simulink model "SLemba_dropTest"  (R2024a)
settings: Solver=FixedStepAuto  StartTime=0.0  StopTime=inf  RelTol=1e-3
InitFcn:
  | busObjects;
libraries: aru_toolbox x1
settings Model: Creator=Mechatronics  LastModifiedBy=Mechatronics
settings SolverCC: ConcurrentTasks=on  PositivePriorityOrder=on
settings OptimizationCC: BlockReduction=off  OptimizeBlockIOStorage=off
settings DebuggingCC: TasksWithSamePriorityMsg=none
settings HardwareCC: ProdBitPerLong=64  ProdLongLongMode=on  ProdHWDeviceType=Intel->x86-64 (Linux 64)
settings RTWCC: Description=Speedgoat Real-Time Target Machine  SystemTargetFile=speedgoat.tlc  TemplateMakefile=slrealtime_default_tmf  Toolchain=Simulink Real-Time Toolchain  BuildConfiguration=Faster Runs  CodeExecutionProfiling=on  TargetLang=C++
settings SimulinkRealTimeTargetCC: InstructionSetFMA=off  LogToMDFFile=off

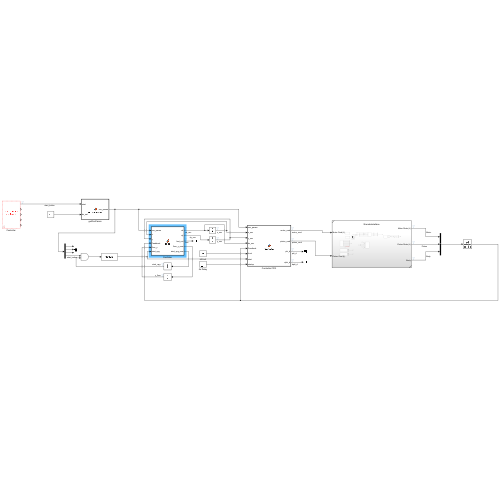
[thumbnail: Simulink's stored preview of the top-level diagram]
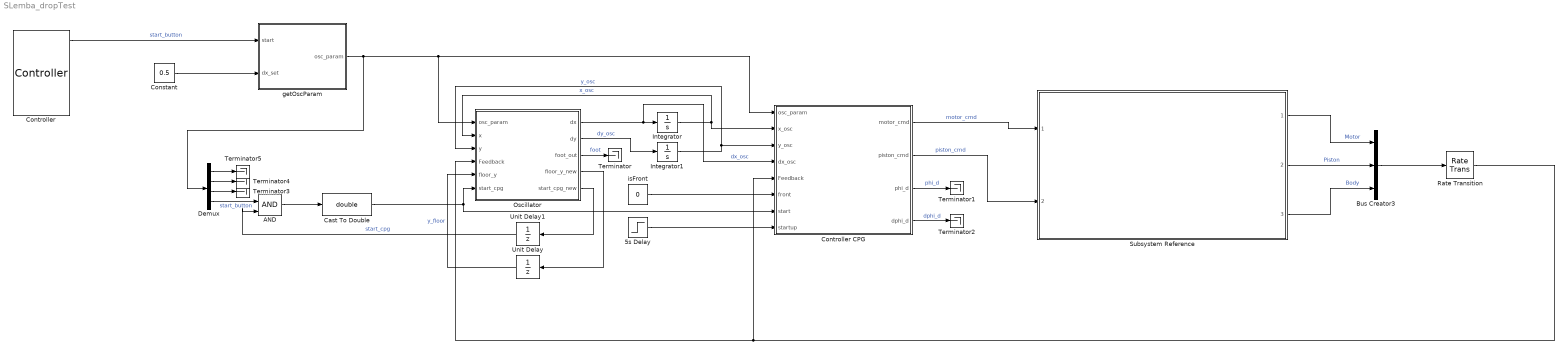
== system SLemba_dropTest ==
  5s Delay : Step  Time=5  SampleTime=0
  AND : Logic  IconShape=distinctive  AllPortsSameDT=off  OutDataTypeStr=boolean
  Bus Creator3 : BusCreator  Inputs=3  OutDataTypeStr=Bus: State  NonVirtualBus=on
      settings: InheritFromInputs=off
  Cast To Double : DataTypeConversion  OutDataTypeStr=double  SaturateOnIntegerOverflow=off  RndMeth=Floor
  Constant : Constant  Value=0.5
  Controller : aru_toolbox/Controller
      settings: SourceProductName=ARU Toolbox
  Controller CPG : MATLAB Function  TreatAsAtomicUnit=on
  Demux : Demux
  Integrator : Integrator
  Integrator1 : Integrator  InitialCondition=1
  Oscillator : MATLAB Function  TreatAsAtomicUnit=on
  Rate Transition : RateTransition
  Subsystem Reference : Subsystem  ReferencedSubsystem=SLembaInterface
  Terminator{,1..5} (6 alike) : Terminator
  Unit Delay : UnitDelay  SampleTime=-1  HasFrameUpgradeWarning=on
  Unit Delay1 : UnitDelay  SampleTime=-1  HasFrameUpgradeWarning=on
  getOscParam : MATLAB Function  TreatAsAtomicUnit=on
  isFront : Constant  Value=0
  wires:
  Subsystem Reference/1 -> Bus Creator3/1  "Motor"
  Subsystem Reference/2 -> Bus Creator3/2  "Piston"
  Subsystem Reference/3 -> Bus Creator3/3  "Body"
  Oscillator/4(floor_y_new) -> Unit Delay/1
  Unit Delay/1 -> Oscillator/5(floor_y)  "y_floor"
  Oscillator/5(start_cpg_new) -> Unit Delay1/1
  Oscillator/3(foot_out) -> Terminator/1  "foot"
  Oscillator/1(dx) -> Integrator/1, Controller CPG/4(dx_osc)  "dx_osc"
  Oscillator/2(dy) -> Integrator1/1  "dy_osc"
  Integrator/1 -> Controller CPG/2(x_osc), Oscillator/2(x)  "x_osc"
  Integrator1/1 -> Controller CPG/3(y_osc), Oscillator/3(y)  "y_osc"
  getOscParam/1(osc_param) -> Demux/1, Oscillator/1(osc_param), Controller CPG/1(osc_param)
  isFront/1 -> Controller CPG/6(front)
  Controller CPG/1(motor_cmd) -> Subsystem Reference/1  "motor_cmd"
  Controller CPG/2(piston_cmd) -> Subsystem Reference/2  "piston_cmd"
  Controller CPG/3(phi_d) -> Terminator1/1  "phi_d"
  Controller CPG/4(dphi_d) -> Terminator2/1  "dphi_d"
  Constant/1 -> getOscParam/2(dx_set)
  5s Delay/1 -> Controller CPG/8(startup)
  Bus Creator3/1 -> Rate Transition/1
  Rate Transition/1 -> Controller CPG/5(Feedback), Oscillator/4(Feedback)
  Unit Delay1/1 -> AND/2  "start_cpg"
  AND/1 -> Cast To Double/1
  Cast To Double/1 -> Controller CPG/7(start), Oscillator/6(start_cpg)
  Demux/4 -> AND/1  "start_button"
  Controller/1 -> getOscParam/1(start)  "start_button"
  Demux/3 -> Terminator3/1
  Demux/2 -> Terminator4/1
  Demux/1 -> Terminator5/1

== matlab function SLemba_dropTest/getOscParam ==
  data: osc_param output; start input; dx_set input
function osc_param = osc_paramCalc(start,dx_set) %tst_sol, kx_sol, tsw_sol,

% persistent osc_paramVal
% 
% if isempty(osc_paramVal)
%     out = load("PSO_runs/sol.mat");
%     out = out.out;
%     tst = out.simParams.tst;
%     kx = out.simParams.kx;
% 
%     tsw = out.out.BestSol.Position(4);
% 
%     osc_paramVal = [tst,tsw,kx];
% end

persistent state % 0 is wait, 1 is green button pressed to start

if isempty(state)
    state = 0;
end

switch(state)
    case 0
        if(start)
            state = 1;
        end
end
   

tst = 0;
kx = 0;
tsw = 0;

if state
    dx = dx_set;
    
    % tst = polyval(tst_sol,dx);
    % kx = polyval(kx_sol,dx);
    % tsw = polyval(tsw_sol,dx);

    tst = 0.08;
    kx = 0.15;
    tsw = 0.33;

    % tst = 1;
    % kx = 0.15;
    % tsw = 2;
end

osc_param = [tst,tsw,kx,state];

== matlab function SLemba_dropTest/Controller CPG ==
  settings: updateMethod=DISCRETE
  data: motor_cmd output Bus: MotorCmd; osc_param input; x_osc input; piston_cmd output Bus: PistonCmd; y_osc input; dx_osc input; Feedback input; front input; phi_d output; dphi_d output; start input; startup input
function [motor_cmd,piston_cmd,phi_d,dphi_d] = Controller(osc_param, x_osc,y_osc,dx_osc,Feedback,front, start, startup)

persistent state_control % 1 = wait, 2 = startup, 3 = stop

if isempty(state_control)
    state_control = 1;
end

motor_state = Feedback.Motor; piston_state = Feedback.Piston;

kx = osc_param(3);

l = piston_state.p;
dl = piston_state.v;
th = motor_state.q;

if (front)
    direction = -1;
else
    direction = 1;
end

% set command
phi_d = direction*x_osc*kx + pi/2;
dphi_d = direction*dx_osc*kx;
if (y_osc>=0) 
    if(x_osc>=0)
        ue = 0; ur = 1;
    else
            ue = 1; ur = 1;
    end
else
    ue = 1; ur = 0;
end

kp = 250;
kd = 10;

% % Testing
% % ----------
% ue = 1; ur = 0;
% phi_d = pi/2; dphi_d = 0;
% kp = 250;kd = 5;
% % ---------

if start == 0
    ue = 0; ur = 1;
    phi_d = pi/2; dphi_d = 0;
end

switch(state_control)
    case 1
        if startup == 1
            state_control = 2;
        end
    case 2
        if y_osc<0
            state_control = 3;
        end
end

switch(state_control)
    case 2
        piston_cmd.ue = ue;
        piston_cmd.ur = ur;
        
        motor_cmd.q = th_calc(phi_d,l);
        motor_cmd.w = dth_calc(phi_calc(th,l),l,dphi_d,dl);
        motor_cmd.Kp = kp;
        motor_cmd.Kd = kd;
        motor_cmd.tff = 0;
    case 3
        piston_cmd.ue = 1;
        piston_cmd.ur = 1;
        
        motor_cmd.q = th_calc(pi/2,l);
        motor_cmd.w = 0;
        motor_cmd.Kp = 100;
        motor_cmd.Kd = 4;
        motor_cmd.tff = 0;
    otherwise
        piston_cmd.ue = 0;
        piston_cmd.ur = 0;
        
        motor_cmd.q = 0;
        motor_cmd.w = 0;
        motor_cmd.Kp = 0;
        motor_cmd.Kd = 0;
        motor_cmd.tff = 0;
end

== matlab function SLemba_dropTest/Oscillator ==
  data: osc_param input; x input size=1; dx output size=1; y input; Feedback input; dy output; foot_out output; floor_y_new output; floor_y input; start_cpg input; start_cpg_new output
% function [dx,dy,floor_y_new,foot_out,start_cpg_new] = CPG(x,y,Body_state,Piston_state, Motor_state, osc_param,floor_y,start,start_cpg)%,dy_lift, fit)%dq_osc = CPG(input_osc)%
% x = input_osc.x_osc; y = input_osc.y_osc; osc_param = input_osc.osc_param;
% Body_state = input_osc.Body_state; Piston_state = input_osc.Piston_state; Motor_state = input_osc.Motor_state;
function [dx,dy,foot_out,floor_y_new,start_cpg_new] = CPG(osc_param,x,y,Feedback, floor_y,start_cpg)%,dy_lift, fit)%dq_osc = CPG(input_osc)%

Body_state = Feedback.Body; Motor_state = Feedback.Motor; Piston_state = Feedback.Piston;

x_body = Body_state.x; y_body = Body_state.y;
dx_body = Body_state.dx; dy_body = Body_state.dy;
th = Motor_state.q; dth = Motor_state.w;
l = Piston_state.p; dl = Piston_state.v;

thk = thk_calc(th,l); tha = tha_calc(th,l);
dthk = dthk_calc(th,l,dth,dl); dtha = dtha_calc(th,l,dth,dl);

foot = foot_Func(x_body,y_body,th,l,thk,tha,dx_body,dy_body,dth,dl,dthk,dtha);

y_foot = foot(2);
dy_foot = foot(4);

% % update floor height based on piston impact
% piston_tol = -1.5e2;
% if (Piston_state.a < piston_tol && osc_param(4))
%     floor_y = y_foot;
% end

% start cpg if in correct state once thrown
dy_tol = -0.5;
if(dy_body - dy_tol<0 && osc_param(4))
% if(osc_param(4))
    start_cpg_new = 1;
else
    start_cpg_new = start_cpg;
end

y_foot = y_foot - floor_y;

foot(2) = y_foot;
foot_out = foot;

floor_y_new = floor_y;

tst = osc_param(1);
tsw = osc_param(2);

% constants
mu = 1;
F_1 = 50;
gamma = 10;
b = 100;


% if(dy_lift>0)
%     coeff = fit.coeff;
% 
%     tsw_new = coeff(1) + coeff(2)*tst + coeff(3)*dy_lift + coeff(4)*tst^2 + coeff(5)*tst*dy_lift + coeff(6)*dy_lift^2;
%     if (tsw_new>tst)
%         tsw = tsw_new;
%     end
% end


T = tst + tsw;
d = tsw/T;
% 
% % 3 frequencies with quadrant crossover
% omega_1 = pi/(T*d);
% omega_2 = omega_1;
% omega_3 = pi/(T - T*d);

k = 1; % 2 for extension at half way
e = 0;%0.4;

% 3 frequencies with quadrant crossover
omega_1 = (pi*k - 2*d*e + 2*d*e*k + pi)/(2*T*d*k);
omega_2 = k*omega_1;
omega_3 = (pi*k - 2*d*e + 2*d*e*k + pi)/(T - T*d + T*k - T*d*k);

% polar coordinates
r = sqrt(x^2 + y^2);
th = atan2(y,x);
% th = atan(y/x);
% if (x <= 0)
%     th = pi + atan(y/x);
% end

% 3 frequencies with quadrant cross over
k1 = omega_1/((exp(-b*(x))+1)*(exp(-b*y)+1));
k2 = omega_2/((exp(b*(x))+1)*(exp(-b*y)+1));
k3 = omega_3/(exp(b*y)+1);
omega = k1 + k2 + k3;

f = @(v) 1 + 0.5*cos(v)*tanh(sin(2*v));
f_dash = @(v) cos(v)*cos(2*v)*(sech(sin(2*v)))^2-0.5*sin(v)*tanh(sin(2*v));

% oscillation
dth = omega;
dr = mu*omega*f_dash(th) + gamma*(mu*f(th)-r);

% change in x
dx = dr*cos(th) - r*sin(th)*dth;

if (y_foot <= 0 && y > 0 && x < 0) % fast transition case 1
    u = -F_1;
elseif(y_foot > 0 && y < 0 && x > 0) % fast transition case 3
    u = F_1;
elseif (y < 0 && dy_foot < 0 && y_foot > 0) % slow transition case 2
    u = - omega*x;
else
    u = 0;
end

u = 0;

dy = dr*sin(th) + r*cos(th)*dth + u;

if start_cpg == 0
    dy = 0;
    dx = 0;
end
end
